simulink model "CoreXY_combined_fullfeed_model_XY"  (R2024b)
settings: Solver=VariableStepAuto  StartTime=0.0  StopTime=max(data.Time_ms_)/1000  RelTol=1e-3
undefined symbols (not defined in the file or in its folder): A_X, A_Y, B_X, B_Y, C_X, C_Y, D_X, D_Y, data, Kd_X, Kd_Y, Ki_X, Ki_Y, Kp_X, Kp_Y, N_X, N_Y
libraries: slpidlib x2
settings Model: Creator=trent  LastModifiedBy=mauro
settings SolverCC: ZeroCrossAlgorithm=Adaptive
settings OptimizationCC: ReuseModelBlockBuffer=off
settings DebuggingCC: IgnoredZcDiagnostic=none  UnconnectedInputMsg=warning  UnconnectedOutputMsg=warning  UnconnectedLineMsg=warning
settings ModelReferenceCC: EnableRefExpFcnMdlSchedulingChecks=on
settings RTWCC: GPUComputeCapability=3.5  DLArmComputeVersion=19.05

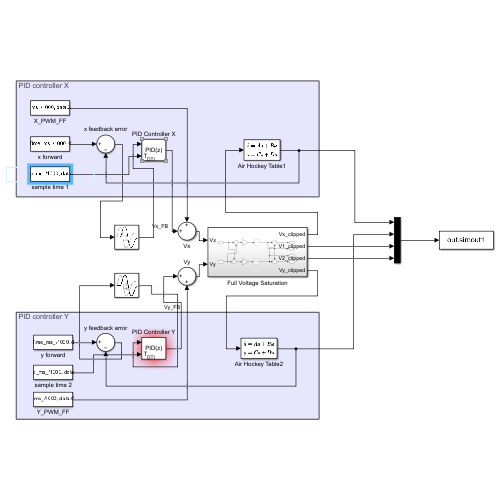
[thumbnail: Simulink's stored preview of the top-level diagram]
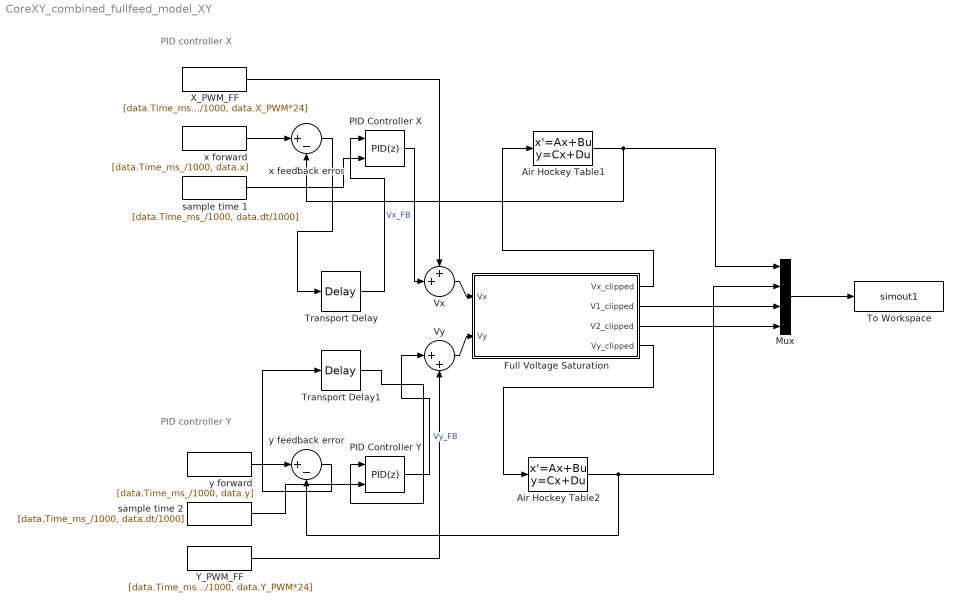
== system CoreXY_combined_fullfeed_model_XY ==
  note: PID controller X
  note: PID controller Y
  Air Hockey Table1 : StateSpace  A=A_X  B=B_X  C=C_X  D=D_X  InitialCondition=[data.X_Accel_m_s2_(1)/C_X(1,3);data.X_Velocity_m_s_(1)/C_X(1,3);data.x(1)/C_X(1,3)]
  Air Hockey Table2 : StateSpace  A=A_Y  B=B_Y  C=C_Y  D=D_Y  InitialCondition=[data.Y_Accel_m_s2_(1)/C_Y(1,3);data.Y_Velocity_m_s_(1)/C_Y(1,3);data.y(1)/C_Y(1,3)]
  Full Voltage Saturation : Subsystem
  Mux : Mux
  PID Controller X : slpidlib/PID Controller  Controller=PID  Form=Parallel  TimeDomain=Discrete-time  UseExternalTs=on  SampleTime=0.35117/1000  IntegratorMethod=Backward Euler  FilterMethod=Backward Euler  ControllerParametersSource=internal  P=Kp_X  I=Ki_X  UseKiTs=off  D=Kd_X  UseExternalDerivativeSource=off  N=N_X  UseFilter=on  TunerSelectOption=Transfer Function Based (PID Tuner App)  InitialConditionSource=internal  InitialConditionForIntegrator=0  InitialConditionForFilter=0  DifferentiatorICPrevScaledInput=0  ExternalReset=none  TrackingMode=off  Kt=1  LimitOutput=off  SatLimitsSource=internal  UpperSaturationLimit=48  LowerSaturationLimit=-48  LinearizeAsGain=on  AntiWindupMode=none  Kb=1  LimitIntegrator=off  UpperIntegratorSaturationLimit=inf  LowerIntegratorSaturationLimit=-inf  POutMin=[]  POutMax=[]  IOutMin=[]  IOutMax=[]  DOutMin=[]  DOutMax=[]  NOutMin=[]  NOutMax=[]  SumOutMin=[]  SumOutMax=[]  SaturationOutMin=[]  SaturationOutMax=[]  PParamMin=[]  PParamMax=[]  IParamMin=[]  IParamMax=[]  DParamMin=[]  DParamMax=[]  NParamMin=[]  NParamMax=[]  KbParamMin=[]  KbParamMax=[]  KtParamMin=[]  KtParamMax=[]  KbOutMin=[]  KbOutMax=[]  KtOutMin=[]  KtOutMax=[]  IntegratorOutMin=[]  IntegratorOutMax=[]  FilterOutMin=[]  FilterOutMax=[]  SumI1OutMin=[]  SumI1OutMax=[]  SumI2OutMin=[]  SumI2OutMax=[]  SumI3OutMin=[]  SumI3OutMax=[]  SumI4OutMin=[]  SumI4OutMax=[]  SumDOutMin=[]  SumDOutMax=[]  DifferentiatorOutMin=[]  DifferentiatorOutMax=[]  FilterDiffOutCoefMin=[]  FilterDiffOutCoefMax=[]  ReciprocalOutMin=[]  ReciprocalOutMax=[]  SumDenOutMin=[]  SumDenOutMax=[]  SumNumOutMin=[]  SumNumOutMax=[]  DivideOutMin=[]  DivideOutMax=[]  UdiffTsProdOutMin=[]  UdiffTsProdOutMax=[]  NTsProdOutMin=[]  NTsProdOutMax=[]  UintegralTsProdOutMin=[]  UintegralTsProdOutMax=[]  UngainTsProdOutMin=[]  UngainTsProdOutMax=[]  ClampingZeroOutDataTypeStr=Inherit: Inherit via back propagation  ClampingZeroOutMin=[]  ClampingZeroOutMax=[]  FilterDenConstantOutDataTypeStr=Inherit: Inherit via back propagation  FilterDenConstantOutMin=[]  FilterDenConstantOutMax=[]  PCopyOutDataTypeStr=Inherit: Inherit via back propagation  PCopyOutMin=[]  PCopyOutMax=[]  NCopyOutDataTypeStr=Inherit: Inherit via back propagation  NCopyOutMin=[]  NCopyOutMax=[]  IntegratorContinuousStateAttributes=''  IntegratorStateMustResolveToSignalObject=off  IntegratorRTWStateStorageClass=Auto  FilterContinuousStateAttributes=''  FilterStateMustResolveToSignalObject=off  FilterRTWStateStorageClass=Auto  ParallelPVariant=InternalParameters  IdealPVariant=Disabled  IVariant=InternalParameters  DVariant=InternalParameters  IntegratorVariant=Discrete  SatVariant=Disabled  AWVariant=Passthrough  PCopyVariant=Disabled  TRVariant=Disabled  FdbkBlocksVariant=Forward  IdealPFdbkVariant=Disabled  SatFdbkVariant=Disabled  DerivativeFilterVariant=BackwardEulerFilter  NVariant=InternalParameters  NCopyVariant=InternalParameters  FilterICVariant=InternalICsFilter  IntegratorICVariant=InternalICs  ExternalResetVariant=Disabled  TRSumVariant=Passthrough  SumFdbkVariant=Disabled  SumVariant=Sum_PID  TsampFilterVariant=ExternalTs  TsampNgainVariant=Passthrough  TsampIntegralVariant=ExternalTs  ExternalSaturationOutDataTypeStr=Inherit: Same as second input  DerivativeSourceVariant=ErrorSignal  PreIntVariant=InternalPreInt
  PID Controller Y : slpidlib/PID Controller  Controller=PID  Form=Parallel  TimeDomain=Discrete-time  UseExternalTs=on  SampleTime=0.35117/1000  IntegratorMethod=Backward Euler  FilterMethod=Backward Euler  ControllerParametersSource=internal  P=Kp_Y  I=Ki_Y  UseKiTs=off  D=Kd_Y  UseExternalDerivativeSource=off  N=N_Y  UseFilter=on  TunerSelectOption=Transfer Function Based (PID Tuner App)  InitialConditionSource=internal  InitialConditionForIntegrator=0  InitialConditionForFilter=0  DifferentiatorICPrevScaledInput=0  ExternalReset=none  TrackingMode=off  Kt=1  LimitOutput=off  SatLimitsSource=internal  UpperSaturationLimit=48  LowerSaturationLimit=-48  LinearizeAsGain=on  AntiWindupMode=none  Kb=1  LimitIntegrator=off  UpperIntegratorSaturationLimit=inf  LowerIntegratorSaturationLimit=-inf  POutMin=[]  POutMax=[]  IOutMin=[]  IOutMax=[]  DOutMin=[]  DOutMax=[]  NOutMin=[]  NOutMax=[]  SumOutMin=[]  SumOutMax=[]  SaturationOutMin=[]  SaturationOutMax=[]  PParamMin=[]  PParamMax=[]  IParamMin=[]  IParamMax=[]  DParamMin=[]  DParamMax=[]  NParamMin=[]  NParamMax=[]  KbParamMin=[]  KbParamMax=[]  KtParamMin=[]  KtParamMax=[]  KbOutMin=[]  KbOutMax=[]  KtOutMin=[]  KtOutMax=[]  IntegratorOutMin=[]  IntegratorOutMax=[]  FilterOutMin=[]  FilterOutMax=[]  SumI1OutMin=[]  SumI1OutMax=[]  SumI2OutMin=[]  SumI2OutMax=[]  SumI3OutMin=[]  SumI3OutMax=[]  SumI4OutMin=[]  SumI4OutMax=[]  SumDOutMin=[]  SumDOutMax=[]  DifferentiatorOutMin=[]  DifferentiatorOutMax=[]  FilterDiffOutCoefMin=[]  FilterDiffOutCoefMax=[]  ReciprocalOutMin=[]  ReciprocalOutMax=[]  SumDenOutMin=[]  SumDenOutMax=[]  SumNumOutMin=[]  SumNumOutMax=[]  DivideOutMin=[]  DivideOutMax=[]  UdiffTsProdOutMin=[]  UdiffTsProdOutMax=[]  NTsProdOutMin=[]  NTsProdOutMax=[]  UintegralTsProdOutMin=[]  UintegralTsProdOutMax=[]  UngainTsProdOutMin=[]  UngainTsProdOutMax=[]  ClampingZeroOutDataTypeStr=Inherit: Inherit via back propagation  ClampingZeroOutMin=[]  ClampingZeroOutMax=[]  FilterDenConstantOutDataTypeStr=Inherit: Inherit via back propagation  FilterDenConstantOutMin=[]  FilterDenConstantOutMax=[]  PCopyOutDataTypeStr=Inherit: Inherit via back propagation  PCopyOutMin=[]  PCopyOutMax=[]  NCopyOutDataTypeStr=Inherit: Inherit via back propagation  NCopyOutMin=[]  NCopyOutMax=[]  IntegratorContinuousStateAttributes=''  IntegratorStateMustResolveToSignalObject=off  IntegratorRTWStateStorageClass=Auto  FilterContinuousStateAttributes=''  FilterStateMustResolveToSignalObject=off  FilterRTWStateStorageClass=Auto  ParallelPVariant=InternalParameters  IdealPVariant=Disabled  IVariant=InternalParameters  DVariant=InternalParameters  IntegratorVariant=Discrete  SatVariant=Disabled  AWVariant=Passthrough  PCopyVariant=Disabled  TRVariant=Disabled  FdbkBlocksVariant=Forward  IdealPFdbkVariant=Disabled  SatFdbkVariant=Disabled  DerivativeFilterVariant=BackwardEulerFilter  NVariant=InternalParameters  NCopyVariant=InternalParameters  FilterICVariant=InternalICsFilter  IntegratorICVariant=InternalICs  ExternalResetVariant=Disabled  TRSumVariant=Passthrough  SumFdbkVariant=Disabled  SumVariant=Sum_PID  TsampFilterVariant=ExternalTs  TsampNgainVariant=Passthrough  TsampIntegralVariant=ExternalTs  ExternalSaturationOutDataTypeStr=Inherit: Same as second input  DerivativeSourceVariant=ErrorSignal  PreIntVariant=InternalPreInt
  To Workspace : ToWorkspace  VariableName=simout1  SaveFormat=Timeseries  SampleTime=-1
  Transport Delay : TransportDelay  DelayTime=0.00009
  Transport Delay1 : TransportDelay  DelayTime=0.00009
  Vx : Sum  Inputs=++|
  Vy : Sum  Inputs=|++
  X_PWM_FF : FromWorkspace  VariableName=[data.Time_ms_/1000, data.X_PWM*24]
  Y_PWM_FF : FromWorkspace  VariableName=[data.Time_ms_/1000, data.Y_PWM*24]
  sample time 1 : FromWorkspace  VariableName=[data.Time_ms_/1000, data.dt/1000]
  sample time 2 : FromWorkspace  VariableName=[data.Time_ms_/1000, data.dt/1000]
  x feedback error : Sum  Inputs=|+-
  x forward : FromWorkspace  VariableName=[data.Time_ms_/1000, data.x]
  y feedback error : Sum  Inputs=|+-
  y forward : FromWorkspace  VariableName=[data.Time_ms_/1000, data.y]
  wires:
  Air Hockey Table1/1 -> x feedback error/2, Mux/1
  Air Hockey Table2/1 -> y feedback error/2, Mux/2
  PID Controller X/1 -> Vx/2  "Vx_FB"
  PID Controller Y/1 -> Vy/1  "Vy_FB"
  Mux/1 -> To Workspace/1
  X_PWM_FF/1 -> Vx/1
  Full Voltage Saturation/1(Vx_clipped) -> Air Hockey Table1/1
  Y_PWM_FF/1 -> Vy/2
  Full Voltage Saturation/4(Vy_clipped) -> Air Hockey Table2/1
  Vy/1 -> Full Voltage Saturation/2(Vy)
  Vx/1 -> Full Voltage Saturation/1(Vx)
  x feedback error/1 -> Transport Delay/1
  y feedback error/1 -> Transport Delay1/1
  y forward/1 -> y feedback error/1
  x forward/1 -> x feedback error/1
  Full Voltage Saturation/3(V2_clipped) -> Mux/4
  Full Voltage Saturation/2(V1_clipped) -> Mux/3
  sample time 1/1 -> PID Controller X/2
  Transport Delay1/1 -> PID Controller Y/1
  Transport Delay/1 -> PID Controller X/1
  sample time 2/1 -> PID Controller Y/2

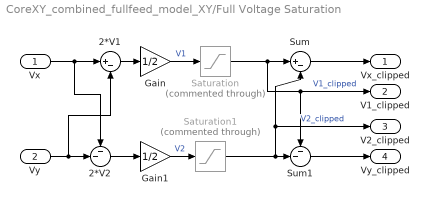
== system CoreXY_combined_fullfeed_model_XY/Full Voltage Saturation ==
  Vx : Inport
  Vy : Inport  Port=2
  2*V1 : Sum  Inputs=|+-
  2*V2 : Sum  Inputs=--|
  Gain : Gain  Gain=1/2
  Gain1 : Gain  Gain=1/2
  Saturation : Saturate  Commented=through  UpperLimit=24  LowerLimit=-24  ZeroCross=off
  Saturation1 : Saturate  Commented=through  UpperLimit=24  LowerLimit=-24  ZeroCross=off
  Sum : Sum  Inputs=|+-
  Sum1 : Sum  Inputs=--|
  Vx_clipped : Outport
  V1_clipped : Outport  Port=2
  V2_clipped : Outport  Port=3
  Vy_clipped : Outport  Port=4
  wires:
  Gain1/1 -> Saturation1/1  "V2"
  Gain/1 -> Saturation/1  "V1"
  Vy/1 -> 2*V1/2, 2*V2/2
  Vx/1 -> 2*V2/1, 2*V1/1
  Saturation1/1 -> Sum1/2, V2_clipped/1, Sum/2  "V2_clipped"
  2*V1/1 -> Gain/1
  Saturation/1 -> Sum/1, V1_clipped/1, Sum1/1  "V1_clipped"
  2*V2/1 -> Gain1/1
  Sum/1 -> Vx_clipped/1
  Sum1/1 -> Vy_clipped/1
